simulink model "cmd_vectorielle_simulink_tri_05"  (R2018b)
settings: Solver=FixedStepAuto  StartTime=0.0  StopTime=Tsim_all  FixedStep=Tid/100  RelTol=1e-3
values from neighbouring files (symbols this model uses):
  Clarke = [2/3 -1/3 -1/3;0 1/sqrt(3) -1/sqrt(3);1/3 1/3 1/3]    [Init_MS.m]
  Cn = Pn*rendn/Wn    (= 4.58366236105)    [Init_MS.m]
  delay_torque = 15    [Init_MS.m]
  fv = 0.0033    [Init_MS.m]
  IClarke = [1 0 1;-1/2 sqrt(3)/2 1;-1/2 -sqrt(3)/2 1]    [Init_MS.m]
  Idref = 0    [Init_MS.m]
  J = 0.05    [Init_MS.m]
  kc = 3/2*p*Phi_f    (= 2.133)    [Init_MS.m]
  Kond = Un/2    [Init_MS.m]
  Kpd = n*Rs/Kond    [Init_MS.m]
  Kpq = n*Rs/Kond    [Init_MS.m]
  kv = 5*fv/kc    (= 0.00773558368495)    [Init_MS.m]
  Ld = 0.245    [Init_MS.m]
  Lq = Ld    (= 0.245)    [Init_MS.m]
  p = 2    [Init_MS.m]
  Phi_f = 0.711    [Init_MS.m]
  Rs = 10.5    [Init_MS.m]
  Tid = Ld/Rs    (= 0.0233333333333)    [Init_MS.m]
  Tiq = Lq/Rs    (= 0.0233333333333)    [Init_MS.m]
  Wn = Nn*2*pi/60    (= 157.079632679)    [Init_MS.m]
libraries: simulink x2
settings Model: Creator=jras  LastModifiedBy=jras
settings DataIOCC: SaveOutput=off  SignalLogging=off  DSMLogging=off  SaveTime=off

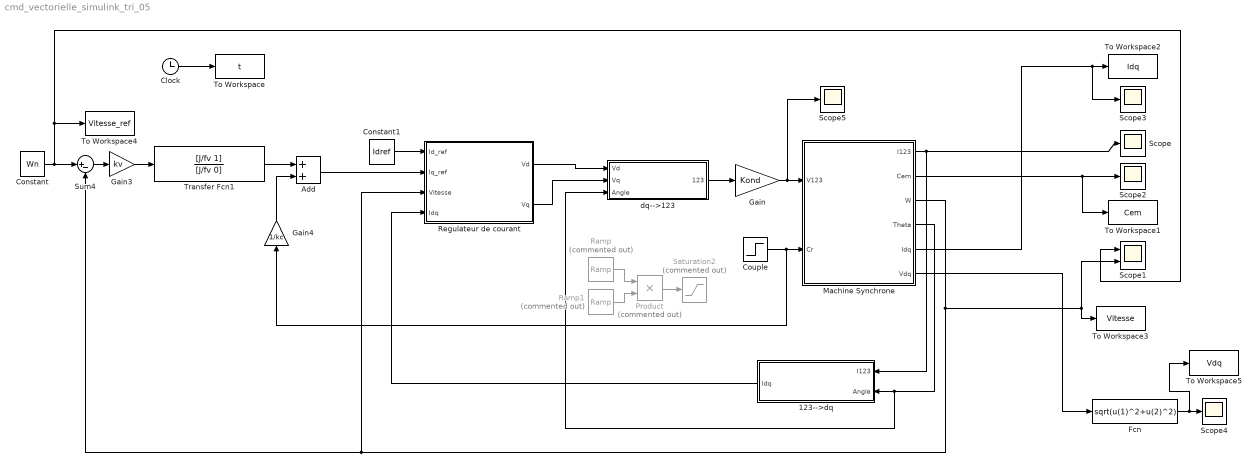
== system cmd_vectorielle_simulink_tri_05 ==
  123-->dq : Subsystem
  Add : Sum
  Clock : Clock
  Constant : Constant  Value=Wn
  Constant1 : Constant  Value=Idref
  Couple : Step  Time=delay_torque  After=Cn  SampleTime=0
  Fcn : Fcn  Expr=sqrt(u(1)^2+u(2)^2)
  Gain : Gain  Gain=Kond
  Gain3 : Gain  Gain=kv
  Gain4 : Gain  Gain=1/kc
  Machine Synchrone : Subsystem
  Product : Product  Commented=on
  Ramp : simulink/Sources/Ramp  Commented=on  slope=0.2  start=delay_torque  InitialOutput=0
  Ramp1 : simulink/Sources/Ramp  Commented=on  slope=0.2  start=delay_torque  InitialOutput=0
  Regulateur de courant : Subsystem
  Saturation2 : Saturate  Commented=on  UpperLimit=Cn  LowerLimit=-Cn
  Scope{,2..5} (5 alike) : Scope
  Scope1 : Scope  NumInputPorts=2
  Sum4 : Sum  Inputs=|+-
  To Workspace : ToWorkspace  VariableName=t  SampleTime=-1
  To Workspace1 : ToWorkspace  VariableName=Cem  SampleTime=-1
  To Workspace2 : ToWorkspace  VariableName=Idq  SampleTime=-1
  To Workspace3 : ToWorkspace  VariableName=Vitesse  SampleTime=-1
  To Workspace4 : ToWorkspace  VariableName=Vitesse_ref  SampleTime=-1
  To Workspace5 : ToWorkspace  VariableName=Vdq  SampleTime=-1
  Transfer Fcn1 : TransferFcn  Numerator=[J/fv 1]  Denominator=[J/fv 0]
  dq-->123 : Subsystem
  wires:
  Machine Synchrone/1(I123) -> Scope/1, 123-->dq/1(I123)
  Machine Synchrone/4(Theta) -> 123-->dq/2(Angle), dq-->123/3(Angle)
  Gain/1 -> Scope5/1, Machine Synchrone/1(V123)
  Machine Synchrone/5(Idq) -> Scope3/1, To Workspace2/1
  Clock/1 -> To Workspace/1
  Machine Synchrone/2(Cem) -> Scope2/1, To Workspace1/1
  Transfer Fcn1/1 -> Add/1
  Constant/1 -> To Workspace4/1, Scope1/1, Sum4/1
  Gain3/1 -> Transfer Fcn1/1
  Sum4/1 -> Gain3/1
  Machine Synchrone/3(W) -> Scope1/2, To Workspace3/1, Regulateur de courant/3(Vitesse), Sum4/2
  Gain4/1 -> Add/2
  Constant1/1 -> Regulateur de courant/1(Id_ref)
  Add/1 -> Regulateur de courant/2(Iq_ref)
  Regulateur de courant/1(Vd) -> dq-->123/1(Vd)
  Regulateur de courant/2(Vq) -> dq-->123/2(Vq)
  dq-->123/1(123) -> Gain/1
  Machine Synchrone/6(Vdq) -> Fcn/1
  Ramp/1 -> Product/1
  Ramp1/1 -> Product/2
  Fcn/1 -> Scope4/1, To Workspace5/1
  Couple/1 -> Machine Synchrone/2(Cr), Gain4/1
  Product/1 -> Saturation2/1
  123-->dq/1(Idq) -> Regulateur de courant/4(Idq)

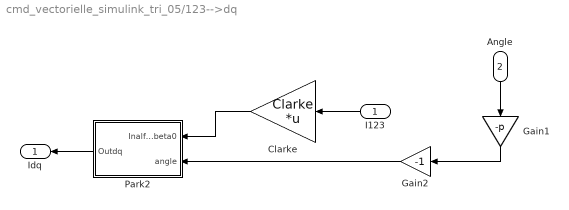
== system cmd_vectorielle_simulink_tri_05/123-->dq ==
  I123 : Inport
  Angle : Inport  Port=2
  Clarke : Gain  Gain=Clarke  Multiplication=Matrix(K*u)
  Gain1 : Gain  Gain=-p
  Gain2 : Gain  Gain=-1
  Park2 : Subsystem
  Idq : Outport
  wires:
  Angle/1 -> Gain1/1
  Gain1/1 -> Gain2/1
  Clarke/1 -> Park2/1(Inalfabeta0)
  Gain2/1 -> Park2/2(angle)
  Park2/1(Outdq) -> Idq/1
  I123/1 -> Clarke/1

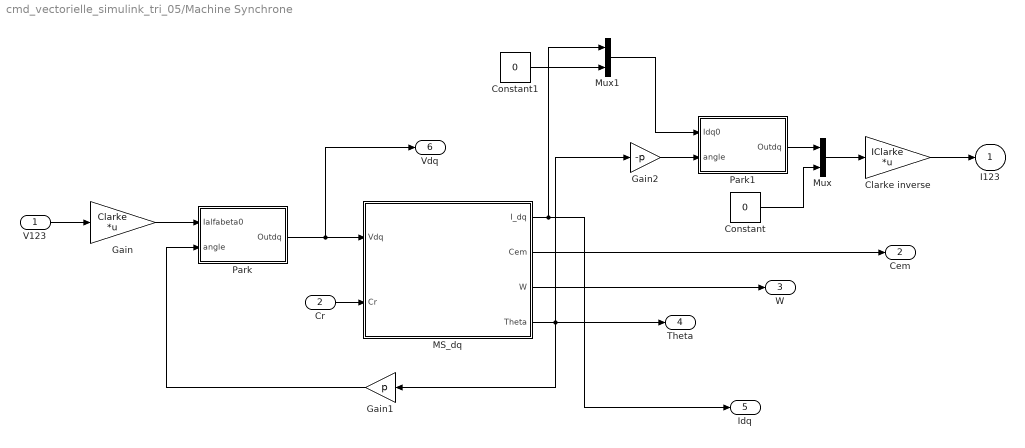
== system cmd_vectorielle_simulink_tri_05/Machine Synchrone ==
  V123 : Inport
  Cr : Inport  Port=2
  Clarke inverse : Gain  Gain=IClarke  Multiplication=Matrix(K*u)
  Constant : Constant  Value=0
  Constant1 : Constant  Value=0
  Gain : Gain  Gain=Clarke  Multiplication=Matrix(K*u)
  Gain1 : Gain  Gain=p
  Gain2 : Gain  Gain=-p
  MS_dq : Subsystem
  Mux : Mux  Inputs=2
  Mux1 : Mux  Inputs=2
  Park : Subsystem
  Park1 : Subsystem
  I123 : Outport
  Cem : Outport  Port=2
  W : Outport  Port=3
  Theta : Outport  Port=4
  Idq : Outport  Port=5
  Vdq : Outport  Port=6
  wires:
  MS_dq/3(W) -> W/1
  MS_dq/1(I_dq) -> Mux1/1, Idq/1
  Cr/1 -> MS_dq/2(Cr)
  MS_dq/4(Theta) -> Gain2/1, Gain1/1, Theta/1
  V123/1 -> Gain/1
  MS_dq/2(Cem) -> Cem/1
  Gain/1 -> Park/1(Ialfabeta0)
  Gain1/1 -> Park/2(angle)
  Gain2/1 -> Park1/2(angle)
  Park1/1(Outdq) -> Mux/1
  Clarke inverse/1 -> I123/1
  Constant/1 -> Mux/2
  Mux/1 -> Clarke inverse/1
  Constant1/1 -> Mux1/2
  Mux1/1 -> Park1/1(Idq0)
  Park/1(Outdq) -> Vdq/1, MS_dq/1(Vdq)

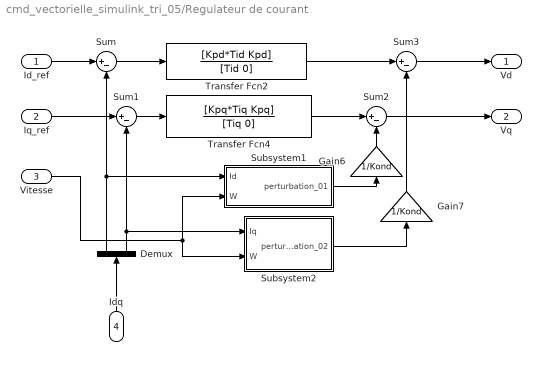
== system cmd_vectorielle_simulink_tri_05/Regulateur de courant ==
  Id_ref : Inport
  Iq_ref : Inport  Port=2
  Vitesse : Inport  Port=3
  Idq : Inport  Port=4
  Demux : Demux  Outputs=2
  Gain6 : Gain  Gain=1/Kond
  Gain7 : Gain  Gain=1/Kond
  Subsystem1 : Subsystem
  Subsystem2 : Subsystem
  Sum{,1..3} (4 alike) : Sum  Inputs=|+-
  Transfer Fcn2 : TransferFcn  Numerator=[Kpd*Tid Kpd]  Denominator=[Tid 0]
  Transfer Fcn4 : TransferFcn  Numerator=[Kpq*Tiq Kpq]  Denominator=[Tiq 0]
  Vd : Outport
  Vq : Outport  Port=2
  wires:
  Demux/1 -> Sum/2, Subsystem1/1(Id)
  Subsystem2/1(perturbation_02) -> Gain7/1
  Gain7/1 -> Sum3/2
  Demux/2 -> Sum1/2, Subsystem2/1(Iq)
  Vitesse/1 -> Subsystem2/2(W), Subsystem1/2(W)
  Sum/1 -> Transfer Fcn2/1
  Iq_ref/1 -> Sum1/1
  Transfer Fcn4/1 -> Sum2/1
  Sum1/1 -> Transfer Fcn4/1
  Transfer Fcn2/1 -> Sum3/1
  Gain6/1 -> Sum2/2
  Subsystem1/1(perturbation_01) -> Gain6/1
  Sum2/1 -> Vq/1
  Sum3/1 -> Vd/1
  Idq/1 -> Demux/1
  Id_ref/1 -> Sum/1

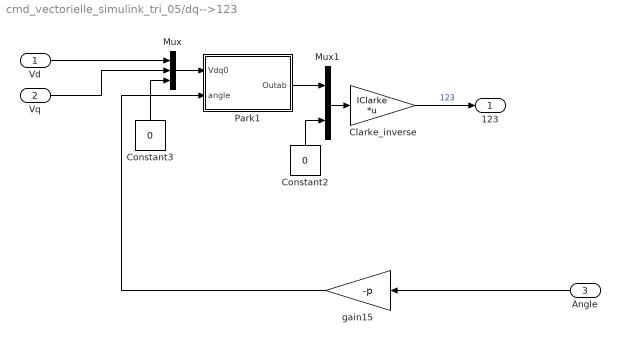
== system cmd_vectorielle_simulink_tri_05/dq-->123 ==
  Vd : Inport
  Vq : Inport  Port=2
  Angle : Inport  Port=3
  Clarke_inverse : Gain  Gain=IClarke  Multiplication=Matrix(K*u)
  Constant2 : Constant  Value=0
  Constant3 : Constant  Value=0
  Mux : Mux  Inputs=3
  Mux1 : Mux  Inputs=2
  Park1 : Subsystem
  gain15 : Gain  Gain=-p
  123 : Outport
  wires:
  Mux/1 -> Park1/1(Vdq0)
  Angle/1 -> gain15/1
  Constant2/1 -> Mux1/2
  Park1/1(Outab) -> Mux1/1
  Mux1/1 -> Clarke_inverse/1
  Vd/1 -> Mux/1
  Clarke_inverse/1 -> 123/1  "123"
  Constant3/1 -> Mux/3
  Vq/1 -> Mux/2
  gain15/1 -> Park1/2(angle)

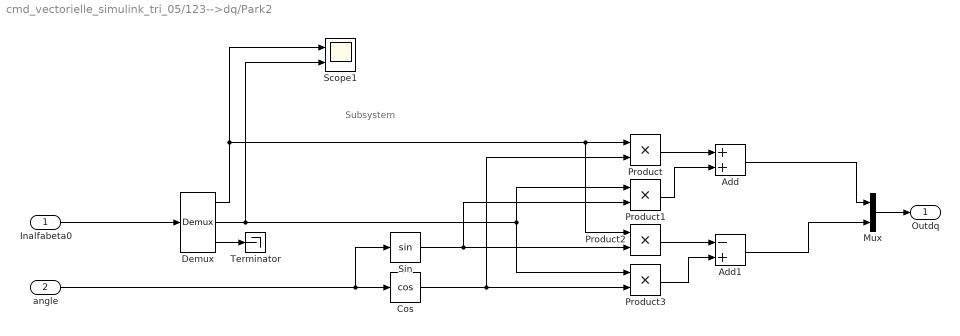
== system cmd_vectorielle_simulink_tri_05/123-->dq/Park2 ==
  note: Subsystem
  Inalfabeta0 : Inport
  angle : Inport  Port=2
  Add : Sum
  Add1 : Sum  Inputs=-+
  Cos : Trigonometry  Operator=cos
  Demux : Demux  Outputs=3
  Mux : Mux  Inputs=2
  Product{,1..3} (4 alike) : Product
  Scope1 : Scope  NumInputPorts=2
  Sin : Trigonometry
  Terminator : Terminator
  Outdq : Outport
  wires:
  Product3/1 -> Add1/2
  Product1/1 -> Add/2
  Sin/1 -> Product2/2, Product1/2
  Cos/1 -> Product3/2, Product/2
  Product/1 -> Add/1
  angle/1 -> Sin/1, Cos/1
  Demux/2 -> Product1/1, Product3/1, Scope1/2
  Demux/1 -> Scope1/1, Product2/1, Product/1
  Demux/3 -> Terminator/1
  Product2/1 -> Add1/1
  Add/1 -> Mux/1
  Add1/1 -> Mux/2
  Inalfabeta0/1 -> Demux/1
  Mux/1 -> Outdq/1

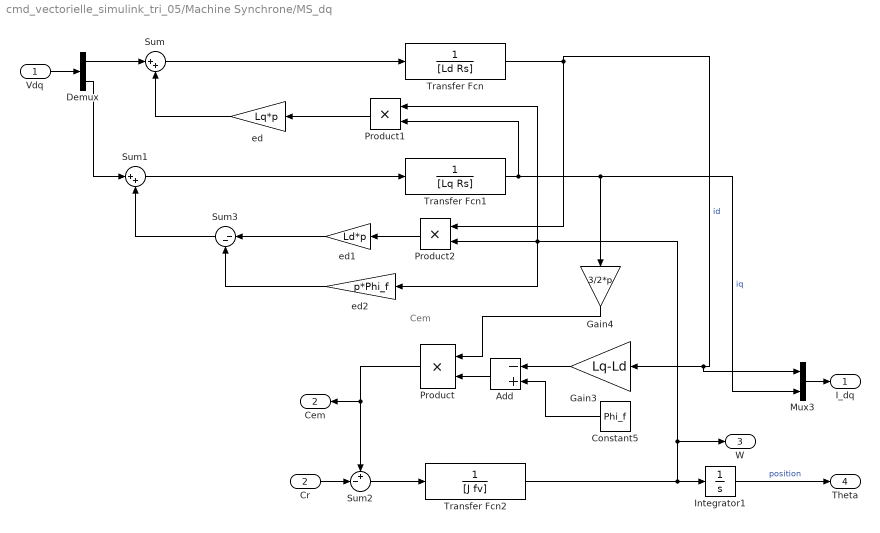
== system cmd_vectorielle_simulink_tri_05/Machine Synchrone/MS_dq ==
  note: Cem
  Vdq : Inport
  Cr : Inport  Port=2
  Add : Sum  Inputs=-+
  Constant5 : Constant  Value=Phi_f
  Demux : Demux  Outputs=2
  Gain3 : Gain  Gain=Lq-Ld
  Gain4 : Gain  Gain=3/2*p
  Integrator1 : Integrator
  Mux3 : Mux  Inputs=2
  Product : Product
  Product1 : Product
  Product2 : Product
  Sum : Sum  Inputs=|++
  Sum1 : Sum  Inputs=|++
  Sum2 : Sum  Inputs=+-|
  Sum3 : Sum  Inputs=|--
  Transfer Fcn : TransferFcn  Denominator=[Ld Rs]
  Transfer Fcn1 : TransferFcn  Denominator=[Lq Rs]
  Transfer Fcn2 : TransferFcn  Denominator=[J fv]
  ed : Gain  Gain=Lq*p
  ed1 : Gain  Gain=Ld*p
  ed2 : Gain  Gain=p*Phi_f
  I_dq : Outport
  Cem : Outport  Port=2
  W : Outport  Port=3
  Theta : Outport  Port=4
  wires:
  Sum/1 -> Transfer Fcn/1
  Transfer Fcn1/1 -> Product1/2, Mux3/2, Gain4/1  "iq"
  Transfer Fcn/1 -> Product2/1, Mux3/1, Gain3/1  "id"
  Sum2/1 -> Transfer Fcn2/1
  Sum1/1 -> Transfer Fcn1/1
  Transfer Fcn2/1 -> Integrator1/1, Product1/1, ed2/1, Product2/2, W/1
  Product/1 -> Sum2/1, Cem/1
  Cr/1 -> Sum2/2
  Integrator1/1 -> Theta/1  "position"
  ed/1 -> Sum/2
  Add/1 -> Product/2
  Constant5/1 -> Add/2
  Gain3/1 -> Add/1
  Product1/1 -> ed/1
  Product2/1 -> ed1/1
  ed1/1 -> Sum3/1
  Sum3/1 -> Sum1/2
  ed2/1 -> Sum3/2
  Gain4/1 -> Product/1
  Mux3/1 -> I_dq/1
  Demux/1 -> Sum/1
  Demux/2 -> Sum1/1
  Vdq/1 -> Demux/1

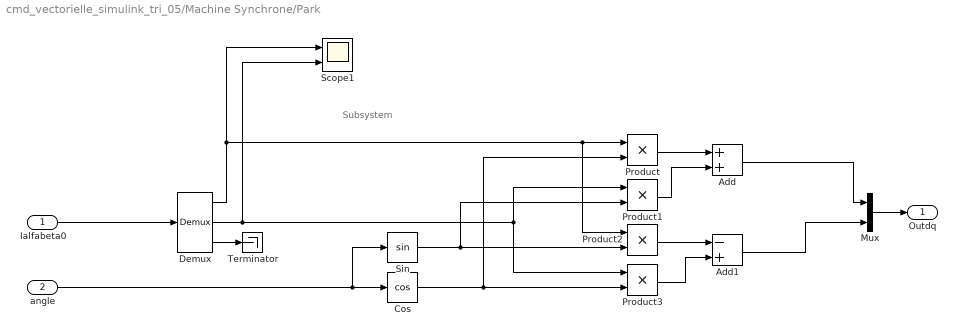
== system cmd_vectorielle_simulink_tri_05/Machine Synchrone/Park ==
  note: Subsystem
  Ialfabeta0 : Inport
  angle : Inport  Port=2
  Add : Sum
  Add1 : Sum  Inputs=-+
  Cos : Trigonometry  Operator=cos
  Demux : Demux  Outputs=3
  Mux : Mux  Inputs=2
  Product{,1..3} (4 alike) : Product
  Scope1 : Scope  NumInputPorts=2
  Sin : Trigonometry
  Terminator : Terminator
  Outdq : Outport
  wires:
  Product3/1 -> Add1/2
  Product1/1 -> Add/2
  Sin/1 -> Product2/2, Product1/2
  Cos/1 -> Product3/2, Product/2
  Product/1 -> Add/1
  angle/1 -> Sin/1, Cos/1
  Demux/2 -> Product1/1, Product3/1, Scope1/2
  Demux/1 -> Scope1/1, Product2/1, Product/1
  Demux/3 -> Terminator/1
  Product2/1 -> Add1/1
  Add/1 -> Mux/1
  Add1/1 -> Mux/2
  Ialfabeta0/1 -> Demux/1
  Mux/1 -> Outdq/1

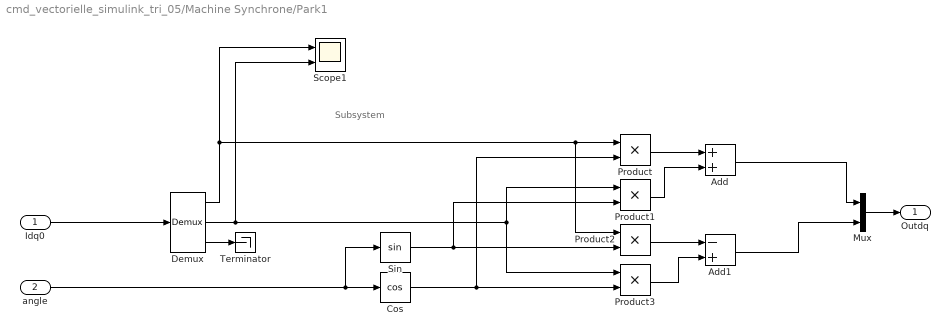
== system cmd_vectorielle_simulink_tri_05/Machine Synchrone/Park1 ==
  note: Subsystem
  Idq0 : Inport
  angle : Inport  Port=2
  Add : Sum
  Add1 : Sum  Inputs=-+
  Cos : Trigonometry  Operator=cos
  Demux : Demux  Outputs=3
  Mux : Mux  Inputs=2
  Product{,1..3} (4 alike) : Product
  Scope1 : Scope  NumInputPorts=2
  Sin : Trigonometry
  Terminator : Terminator
  Outdq : Outport
  wires:
  Mux/1 -> Outdq/1
  Idq0/1 -> Demux/1
  Add1/1 -> Mux/2
  Add/1 -> Mux/1
  Product2/1 -> Add1/1
  Demux/3 -> Terminator/1
  Demux/1 -> Product/1, Product2/1, Scope1/1
  Demux/2 -> Scope1/2, Product3/1, Product1/1
  angle/1 -> Cos/1, Sin/1
  Product/1 -> Add/1
  Cos/1 -> Product/2, Product3/2
  Sin/1 -> Product1/2, Product2/2
  Product1/1 -> Add/2
  Product3/1 -> Add1/2

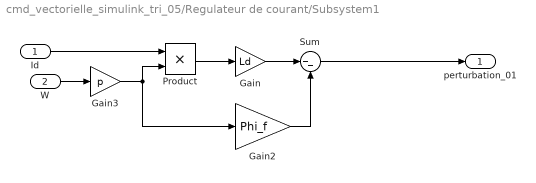
== system cmd_vectorielle_simulink_tri_05/Regulateur de courant/Subsystem1 ==
  Id : Inport
  W : Inport  Port=2
  Gain : Gain  Gain=Ld
  Gain2 : Gain  Gain=Phi_f
  Gain3 : Gain  Gain=p
  Product : Product
  Sum : Sum  Inputs=|--
  perturbation_01 : Outport
  wires:
  Id/1 -> Product/1
  Product/1 -> Gain/1
  Gain/1 -> Sum/1
  Sum/1 -> perturbation_01/1
  Gain2/1 -> Sum/2
  W/1 -> Gain3/1
  Gain3/1 -> Product/2, Gain2/1

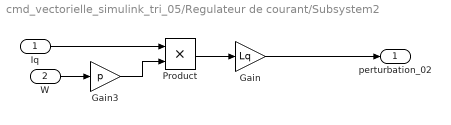
== system cmd_vectorielle_simulink_tri_05/Regulateur de courant/Subsystem2 ==
  Iq : Inport
  W : Inport  Port=2
  Gain : Gain  Gain=Lq
  Gain3 : Gain  Gain=p
  Product : Product
  perturbation_02 : Outport
  wires:
  Gain3/1 -> Product/2
  W/1 -> Gain3/1
  Gain/1 -> perturbation_02/1
  Product/1 -> Gain/1
  Iq/1 -> Product/1

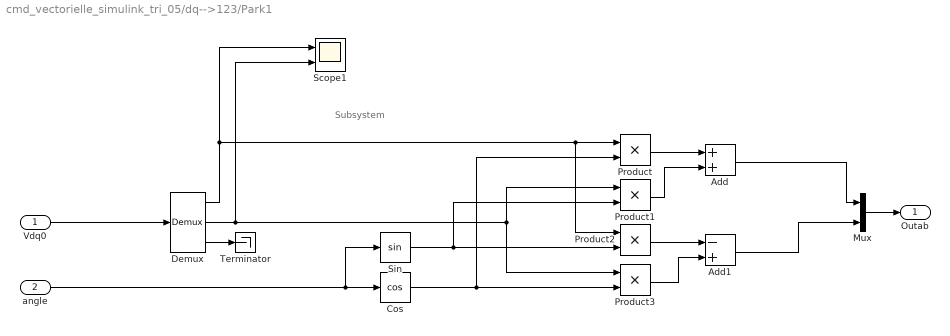
== system cmd_vectorielle_simulink_tri_05/dq-->123/Park1 ==
  note: Subsystem
  Vdq0 : Inport
  angle : Inport  Port=2
  Add : Sum
  Add1 : Sum  Inputs=-+
  Cos : Trigonometry  Operator=cos
  Demux : Demux  Outputs=3
  Mux : Mux  Inputs=2
  Product{,1..3} (4 alike) : Product
  Scope1 : Scope  NumInputPorts=2
  Sin : Trigonometry
  Terminator : Terminator
  Outab : Outport
  wires:
  Mux/1 -> Outab/1
  Vdq0/1 -> Demux/1
  Add1/1 -> Mux/2
  Add/1 -> Mux/1
  Product2/1 -> Add1/1
  Demux/3 -> Terminator/1
  Demux/1 -> Product/1, Product2/1, Scope1/1
  Demux/2 -> Scope1/2, Product3/1, Product1/1
  angle/1 -> Cos/1, Sin/1
  Product/1 -> Add/1
  Cos/1 -> Product/2, Product3/2
  Sin/1 -> Product1/2, Product2/2
  Product1/1 -> Add/2
  Product3/1 -> Add1/2
